simulink model "aluna_pbr_simulink"  (R2026a)
settings: Solver=ode45  StopTime=72.0  MaxStep=0.05
settings Model: Creator=jhon  LastModifiedBy=jhon

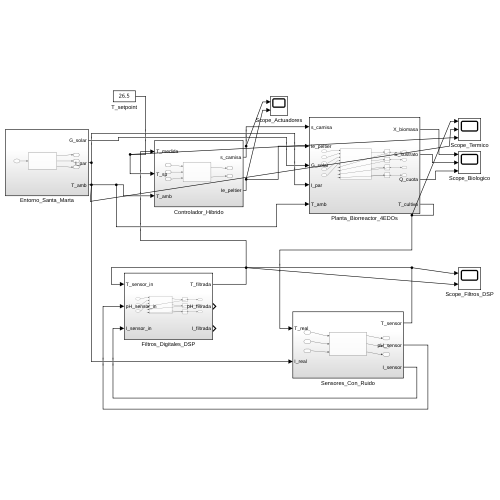
[thumbnail: Simulink's stored preview of the top-level diagram]
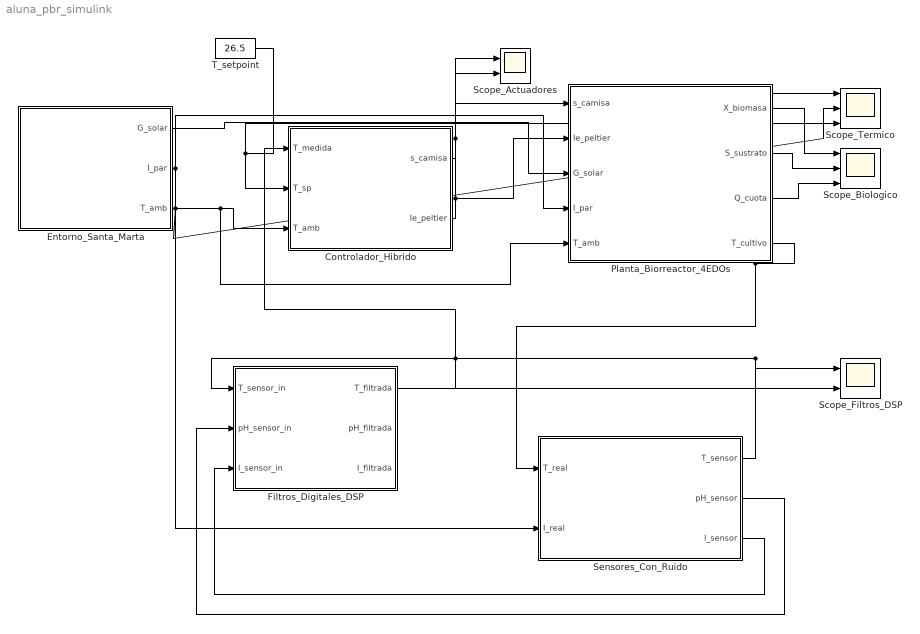
== system aluna_pbr_simulink ==
  Controlador_Hibrido : Subsystem
  Entorno_Santa_Marta : Subsystem
  Filtros_Digitales_DSP : Subsystem
  Planta_Biorreactor_4EDOs : Subsystem
  Scope_Actuadores : Scope  NumInputPorts=2
      settings: ActiveDisplayYMinimum=-0.18749999999999994  ActiveDisplayYMaximum=1.6875
  Scope_Biologico : Scope  NumInputPorts=3
      settings: ActiveDisplayYMinimum=-1.7970752565735668  ActiveDisplayYMaximum=16.173677309162105
  Scope_Filtros_DSP : Scope  NumInputPorts=2
      settings: ActiveDisplayYMinimum=25.05645284655316  ActiveDisplayYMaximum=28.84730181941266
  Scope_Termico : Scope  NumInputPorts=3
      settings: ActiveDisplayYMinimum=23.875000046615071  ActiveDisplayYMaximum=35.124999580918093
  Sensores_Con_Ruido : Subsystem
  T_setpoint : Constant  Value=26.5
  wires:
  Entorno_Santa_Marta/1(G_solar) -> Planta_Biorreactor_4EDOs/3(G_solar)
  Entorno_Santa_Marta/2(I_par) -> Planta_Biorreactor_4EDOs/4(I_par), Sensores_Con_Ruido/2(I_real)
  Entorno_Santa_Marta/3(T_amb) -> Planta_Biorreactor_4EDOs/5(T_amb), Controlador_Hibrido/3(T_amb), Scope_Termico/2
  T_setpoint/1 -> Controlador_Hibrido/2(T_sp), Scope_Termico/3
  Controlador_Hibrido/1(s_camisa) -> Planta_Biorreactor_4EDOs/1(s_camisa), Scope_Actuadores/1
  Controlador_Hibrido/2(Ie_peltier) -> Planta_Biorreactor_4EDOs/2(Ie_peltier), Scope_Actuadores/2
  Planta_Biorreactor_4EDOs/4(T_cultivo) -> Sensores_Con_Ruido/1(T_real), Scope_Termico/1
  Sensores_Con_Ruido/1(T_sensor) -> Filtros_Digitales_DSP/1(T_sensor_in), Scope_Filtros_DSP/1
  Sensores_Con_Ruido/2(pH_sensor) -> Filtros_Digitales_DSP/2(pH_sensor_in)
  Sensores_Con_Ruido/3(I_sensor) -> Filtros_Digitales_DSP/3(I_sensor_in)
  Filtros_Digitales_DSP/1(T_filtrada) -> Controlador_Hibrido/1(T_medida), Scope_Filtros_DSP/2
  Planta_Biorreactor_4EDOs/1(X_biomasa) -> Scope_Biologico/1
  Planta_Biorreactor_4EDOs/2(S_sustrato) -> Scope_Biologico/2
  Planta_Biorreactor_4EDOs/3(Q_cuota) -> Scope_Biologico/3

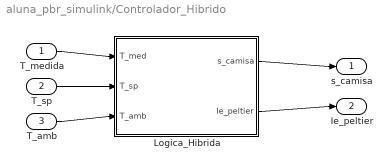
== system aluna_pbr_simulink/Controlador_Hibrido ==
  T_medida : Inport
  T_sp : Inport  Port=2
  T_amb : Inport  Port=3
  Logica_Hibrida : MATLAB Function  TreatAsAtomicUnit=on
  s_camisa : Outport
  Ie_peltier : Outport  Port=2
  wires:
  T_medida/1 -> Logica_Hibrida/1(T_med)
  T_sp/1 -> Logica_Hibrida/2(T_sp)
  T_amb/1 -> Logica_Hibrida/3(T_amb)
  Logica_Hibrida/1(s_camisa) -> s_camisa/1
  Logica_Hibrida/2(Ie_peltier) -> Ie_peltier/1

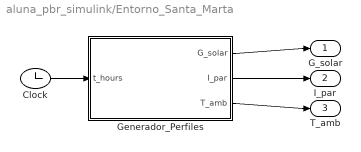
== system aluna_pbr_simulink/Entorno_Santa_Marta ==
  Clock : Clock
  Generador_Perfiles : MATLAB Function  TreatAsAtomicUnit=on
  G_solar : Outport
  I_par : Outport  Port=2
  T_amb : Outport  Port=3
  wires:
  Clock/1 -> Generador_Perfiles/1(t_hours)
  Generador_Perfiles/1(G_solar) -> G_solar/1
  Generador_Perfiles/2(I_par) -> I_par/1
  Generador_Perfiles/3(T_amb) -> T_amb/1

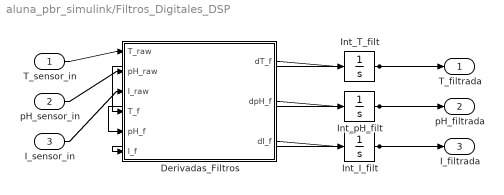
== system aluna_pbr_simulink/Filtros_Digitales_DSP ==
  T_sensor_in : Inport
  pH_sensor_in : Inport  Port=2
  I_sensor_in : Inport  Port=3
  Derivadas_Filtros : MATLAB Function  TreatAsAtomicUnit=on
  Int_I_filt : Integrator  InitialCondition=0.0
  Int_T_filt : Integrator  InitialCondition=28.0
  Int_pH_filt : Integrator  InitialCondition=7.6
  T_filtrada : Outport
  pH_filtrada : Outport  Port=2
  I_filtrada : Outport  Port=3
  wires:
  T_sensor_in/1 -> Derivadas_Filtros/1(T_raw)
  pH_sensor_in/1 -> Derivadas_Filtros/2(pH_raw)
  I_sensor_in/1 -> Derivadas_Filtros/3(I_raw)
  Derivadas_Filtros/1(dT_f) -> Int_T_filt/1
  Derivadas_Filtros/2(dpH_f) -> Int_pH_filt/1
  Derivadas_Filtros/3(dI_f) -> Int_I_filt/1
  Int_T_filt/1 -> T_filtrada/1, Derivadas_Filtros/4(T_f)
  Int_pH_filt/1 -> pH_filtrada/1, Derivadas_Filtros/5(pH_f)
  Int_I_filt/1 -> I_filtrada/1, Derivadas_Filtros/6(I_f)

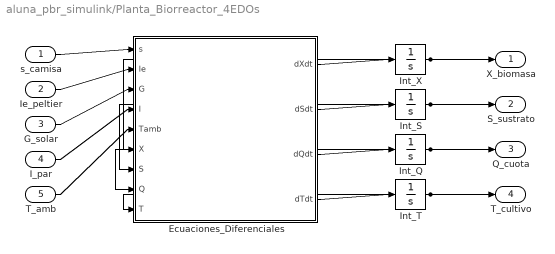
== system aluna_pbr_simulink/Planta_Biorreactor_4EDOs ==
  s_camisa : Inport
  Ie_peltier : Inport  Port=2
  G_solar : Inport  Port=3
  I_par : Inport  Port=4
  T_amb : Inport  Port=5
  Ecuaciones_Diferenciales : MATLAB Function  TreatAsAtomicUnit=on
  Int_Q : Integrator  InitialCondition=5.0  LimitOutput=on  LowerSaturationLimit=1.0
  Int_S : Integrator  InitialCondition=5.0  LimitOutput=on  LowerSaturationLimit=0.0
  Int_T : Integrator  InitialCondition=28.0  LimitOutput=on  UpperSaturationLimit=50.0  LowerSaturationLimit=5.0
  Int_X : Integrator  InitialCondition=0.5  LimitOutput=on  LowerSaturationLimit=1e-6
  X_biomasa : Outport
  S_sustrato : Outport  Port=2
  Q_cuota : Outport  Port=3
  T_cultivo : Outport  Port=4
  wires:
  s_camisa/1 -> Ecuaciones_Diferenciales/1(s)
  Ie_peltier/1 -> Ecuaciones_Diferenciales/2(Ie)
  G_solar/1 -> Ecuaciones_Diferenciales/3(G)
  I_par/1 -> Ecuaciones_Diferenciales/4(I)
  T_amb/1 -> Ecuaciones_Diferenciales/5(Tamb)
  Ecuaciones_Diferenciales/1(dXdt) -> Int_X/1
  Ecuaciones_Diferenciales/2(dSdt) -> Int_S/1
  Ecuaciones_Diferenciales/3(dQdt) -> Int_Q/1
  Ecuaciones_Diferenciales/4(dTdt) -> Int_T/1
  Int_X/1 -> X_biomasa/1, Ecuaciones_Diferenciales/6(X)
  Int_S/1 -> S_sustrato/1, Ecuaciones_Diferenciales/7(S)
  Int_Q/1 -> Q_cuota/1, Ecuaciones_Diferenciales/8(Q)
  Int_T/1 -> T_cultivo/1, Ecuaciones_Diferenciales/9(T)

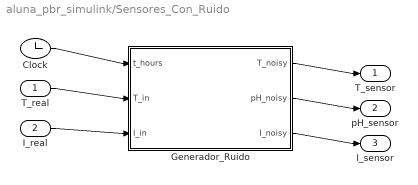
== system aluna_pbr_simulink/Sensores_Con_Ruido ==
  T_real : Inport
  I_real : Inport  Port=2
  Clock : Clock
  Generador_Ruido : MATLAB Function  TreatAsAtomicUnit=on
  T_sensor : Outport
  pH_sensor : Outport  Port=2
  I_sensor : Outport  Port=3
  wires:
  Clock/1 -> Generador_Ruido/1(t_hours)
  T_real/1 -> Generador_Ruido/2(T_in)
  I_real/1 -> Generador_Ruido/3(I_in)
  Generador_Ruido/1(T_noisy) -> T_sensor/1
  Generador_Ruido/2(pH_noisy) -> pH_sensor/1
  Generador_Ruido/3(I_noisy) -> I_sensor/1

== matlab function aluna_pbr_simulink/Controlador_Hibrido/Logica_Hibrida ==
  data: T_med input; s_camisa output; T_sp input; T_amb input; Ie_peltier output
function [s_camisa, Ie_peltier] = Logica_Hibrida(T_med, T_sp, T_amb)
% Lógica de control híbrido bio-inspirado del Frailejón
% Transición suave (sigmoide) para eliminar chattering
e = T_med - T_sp;
% 1. Camisa: transición suave con sigmoide empinada
%    sigma ≈ 0 (cerrada/aislada) cuando T_med << T_sp+1
%    sigma ≈ 1 (abierta/disipa)  cuando T_med >> T_sp+1
sigma = 1.0 / (1.0 + exp(-5.0 * (e - 1.0)));
% Solo abrir camisa si conviene (T_amb < T_med)
if T_amb < T_med
    s_camisa = 1.0 - sigma; % sigma alto -> s=0 (abrir)
else
    s_camisa = 1.0; % Siempre cerrada si afuera hace más calor
end
% 2. Peltier proporcional suave con zona muerta
if e > 0.5
    Ie = 1.5 * (e - 0.5);
    Ie_peltier = min(4.0, max(0.0, Ie));
else
    Ie_peltier = 0.0;
end

== matlab function aluna_pbr_simulink/Entorno_Santa_Marta/Generador_Perfiles ==
  data: t_hours input; G_solar output; I_par output; T_amb output
function [G_solar, I_par, T_amb] = Generador_Perfiles(t_hours)
% Perfil ambiental diario de Santa Marta (ciclo 24h)
hora = mod(t_hours, 24);
if hora >= 6 && hora <= 18
    luz = sin(pi * (hora - 6) / 12);
    G_solar = 850 * max(0, luz);
    I_par   = 1000 * max(0, luz);
else
    G_solar = 0.0;
    I_par   = 0.0;
end
% Temperatura ambiente: oscila entre 25°C (noche) y 34°C (mediodía)
T_amb = 29.5 + 4.5 * sin(2*pi*(hora - 9)/24);

== matlab function aluna_pbr_simulink/Planta_Biorreactor_4EDOs/Ecuaciones_Diferenciales ==
  data: s input; dXdt output; Ie input; G input; I input; Tamb input; X input; S input; Q input; T input; dSdt output; dQdt output; dTdt output
function [dXdt, dSdt, dQdt, dTdt] = Ecuaciones_Diferenciales(s, Ie, G, I, Tamb, X, S, Q, T)
% Parámetros biológicos base
mu_max = 1.1; Qmin = 1.0; Iopt = 200.0; Tmin = 10.0; Topt = 28.0; Tmax = 35.0;
rho_max = 2.0; KS = 0.5; kd = 0.005; D = 0.0; Sin = 5.0;
% 1. Factores de Crecimiento
fI = (I / Iopt) * exp(1 - I / Iopt);
if T > Tmin && T < Tmax
    num = (T - Tmax) * (T - Tmin)^2;
    den = (Topt - Tmin) * ((Topt - Tmin)*(T - Topt) - (Topt - Tmax)*(Topt + Tmin - 2*T));
    fT = max(0.0, min(1.0, num / den));
else
    fT = 0.0;
end
mu = mu_max * (1 - Qmin / max(Q, 1.001)) * fI * fT;
rho = rho_max * S / (KS + S);
% 2. Derivadas biológicas
dXdt = (mu - D - kd) * X;
dSdt = D * (Sin - S) - rho * X;
dQdt = rho - mu * Q;
% 3. Balance térmico
C_tot = 8870.0; % [J/K] = rho*V*cp + Cmasa = 998*0.002*4186 + 500
A_exp = 0.04; alpha_s = 0.30;
Q_solar = alpha_s * A_exp * G;
Q_led = 2.0;
Q_met = 0.5 * X * 2.0; % [W] = Qmet_coeff * X * V * 1000
% Coeficiente U segun estado de camisa (valores de parametros_modelo)
U = (s == 0)*9.35 + (s == 1)*3.56;
Q_pared = U * 0.04 * (T - Tamb);
% Evaporación (Dalton simplificada)
psat_T = 610.78 * exp(17.27 * T / (T + 237.3));
psat_A = 610.78 * exp(17.27 * Tamb / (Tamb + 237.3));
dp = max(0.0, psat_T - 0.6 * psat_A);
Q_evap = 1.5e-8 * 0.01 * dp * 2.26e6;
% Peltier TEC1-12706
Q_peltier = 0.05 * (T + 273.15) * Ie - 0.5 * 2.0 * Ie^2 - 0.5 * (T - Tamb);
Q_peltier = max(0.0, Q_peltier);
dTdt = (Q_solar + Q_led + Q_met - Q_pared - Q_evap - Q_peltier) * 3600.0 / C_tot;

== matlab function aluna_pbr_simulink/Sensores_Con_Ruido/Generador_Ruido ==
  data: t_hours input; T_noisy output; T_in input; I_in input; pH_noisy output; I_noisy output
function [T_noisy, pH_noisy, I_noisy] = Generador_Ruido(t_hours, T_in, I_in)
% Generación de perturbaciones y ruido físico sin variables persistentes
t_sec = t_hours * 3600.0;
% 1. Sensor DS18B20: Temperatura + Ruido Gaussiano + 50Hz
T_noisy = T_in + 0.35 * sin(2*pi*13.7*t_sec) + 0.15 * sin(2*pi*50.0*t_sec);
% 2. Electrodo pH-4502C: Dinámica lenta + Outliers por paso de burbujas
pH_base = 7.6 + 0.15 * sin(2*pi*t_sec/180.0);
outlier = 0.0;
if mod(t_sec, 30.0) < 0.3
    outlier = 1.15; % Pico espurio positivo
elseif mod(t_sec, 47.0) < 0.3
    outlier = -0.85; % Pico espurio negativo
end
pH_noisy = pH_base + 0.04 * sin(2*pi*27.3*t_sec) + outlier;
% 3. Sensor de Radiación: Ruido + atenuación por nubes
nube = 1.0;
if (mod(t_sec, 100.0) > 40.0) && (mod(t_sec, 100.0) < 55.0)
    nube = 0.5;
end
I_noisy = max(0.0, (I_in + 25.0 * sin(2*pi*5.3*t_sec)) * nube);

== matlab function aluna_pbr_simulink/Filtros_Digitales_DSP/Derivadas_Filtros ==
  data: T_raw input; dT_f output; pH_raw input; I_raw input; T_f input; pH_f input; I_f input; dpH_f output; dI_f output
function [dT_f, dpH_f, dI_f] = Derivadas_Filtros(T_raw, pH_raw, I_raw, T_f, pH_f, I_f)
% Algoritmos continuos de filtrado DSP equivalentes
% 1. Filtro IIR (EMA, alpha=0.1 -> tau = 0.5 h)
dT_f = (T_raw - T_f) / 0.5;
% 2. Filtro STM No Lineal (Rechazo de Outliers por tasa acotada)
error_ph = pH_raw - pH_f;
rate_lim = max(-0.4, min(0.4, error_ph / 0.05));
dpH_f = rate_lim;
% 3. Filtro Promedio Movil MA (tau = 0.05 h)
dI_f = (I_raw - I_f) / 0.05;
